simulink model "step_input_lqr"  (R2024a)
settings: Solver=VariableStepAuto  StartTime=0.0  StopTime=10.0  RelTol=1e-3
values from neighbouring files (symbols this model uses):
  A = [-1.7, -0.25, 0 ... (first row only)    [main.m]
  B = [7, 0 ... (first row only)    [main.m]
  K = real(R \ B' * P)    [LQR_own.m]    (also in decoupling.m = Bstar\C_star; main.m = real(inv(R)*B_bar'*P); pole_placement.m = Kbar*T)
settings Model: Creator=chint  LastModifiedBy=chint

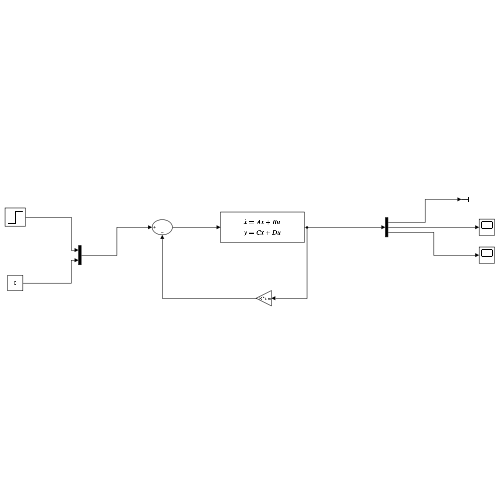
[thumbnail: Simulink's stored preview of the top-level diagram]
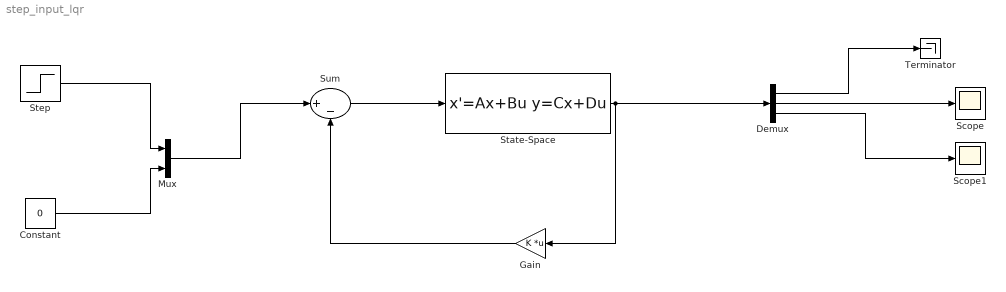
== system step_input_lqr ==
  Constant : Constant  Value=0  VectorParams1D=off
  Demux : Demux  Outputs=3
  Gain : Gain  Gain=K  Multiplication=Matrix(K*u) (u vector)
  Mux : Mux  Inputs=2
  Scope : Scope
  Scope1 : Scope
  State-Space : StateSpace  A=A  B=B  C=eye(3)  D=[0 0; 0 0; 0 0]  InitialCondition=0
  Step : Step  Time=0  SampleTime=0  VectorParams1D=off
  Sum : Sum  Inputs=|+-
  Terminator : Terminator
  wires:
  State-Space/1 -> Demux/1, Gain/1
  Gain/1 -> Sum/2
  Sum/1 -> State-Space/1
  Demux/2 -> Scope/1
  Demux/3 -> Scope1/1
  Demux/1 -> Terminator/1
  Step/1 -> Mux/1
  Constant/1 -> Mux/2
  Mux/1 -> Sum/1
